simulink model "VOO _ONLY"  (R2022b)
settings: Solver=FixedStepAuto  StartTime=0.0  StopTime=10.0  FixedStep=1e-3  RelTol=1e-3  EnableMultiTasking=on
undefined symbols (not defined in the file): D10, D12, D2, D5, D9, PTA2, PTB9, PTC4, PTD0, PTD3
libraries: frdmk64flib x5
settings Model: ExtModeTrigDuration=5  Creator=aldenluscher  LastModifiedBy=aldenluscher
settings OptimizationCC: EnhancedBackFolding=on  PassReuseOutputArgsAs=Individual arguments  ZeroExternalMemoryAtStartup=off  ZeroInternalMemoryAtStartup=off  MaxStackSize=64  OptimizeBlockOrder=speed  DifferentSizesBufferReuse=on  OptimizationCustomize=off  EfficientTunableParamExpr=on
settings DebuggingCC: ParameterTunabilityLossMsg=error
settings HardwareCC: ProdBitPerPointer=32  ProdBitPerSizeT=32  ProdBitPerPtrDiffT=32  ProdLargestAtomicInteger=Long  ProdLargestAtomicFloat=Double  ProdWordSize=32  ProdHWDeviceType=ARM Compatible->ARM Cortex
settings SFSimCC: MATLABDynamicMemAlloc=off
settings RTWCC: Description=Embedded Coder  SystemTargetFile=ert.tlc  HardwareBoard=NXP FRDM-K64F  TLCOptions="-aInlineSetEventsForThisBaseRateFcn=TLC_FALSE -aSuppressMultiTaskScheduler=TLC_FALSE  -aRateBasedStepFcn=0"  TemplateMakefile=ert_default_tmf  Toolchain=GNU Tools for ARM Embedded Processors
settings CodeAppCC: ForceParamTrailComments=on  IgnoreCustomStorageClasses=off  OperatorAnnotations=on  SimulinkDataObjDesc=on  SFDataObjDesc=on  InsertBlockDesc=on
settings ERTTargetCC: ExtModeTransport=4  ExtModeMexFile=sendToCommService

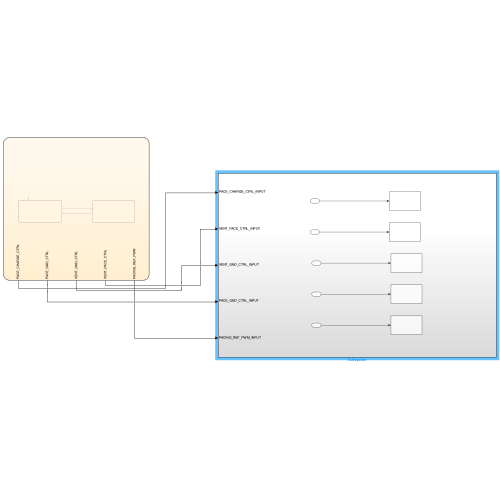
[thumbnail: Simulink's stored preview of the top-level diagram]
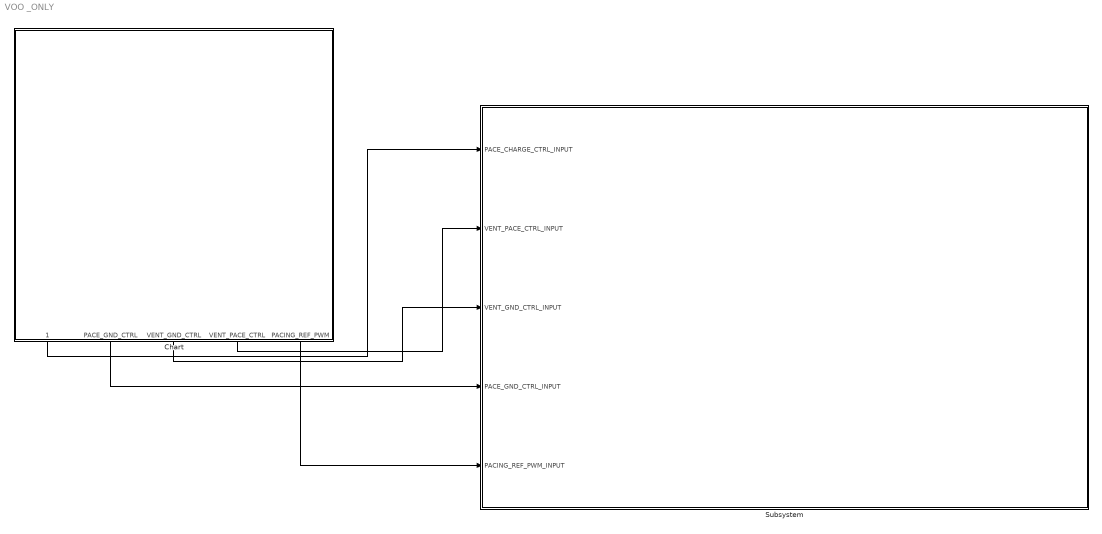
== system VOO _ONLY ==
  Chart : Stateflow chart  TreatAsAtomicUnit=on
      settings: PortSchema="{\"entries\":[{\"content\":{\"sides\":[{\"content\":{\"connectorIds\":[]},\"type\":\"ConnectorPlacement.EquallySpacedRectSide\",\"uuid\":\"ab30f6e3-f4a9-4bd5-815e-4ef92b766934\"},{\"content\":{\"connectorIds\":[],\"side\":\"RIGHT\"},\"type\":\"ConnectorPlacement.EquallySpacedRectSide\",\"uuid\":\"1d0d5e4f-590d-4361-90fd-546c5207ab80\"},{\"content\":{\"connectorIds\":[],\"side\":\"TOP\"},\"type\":\"ConnectorPlacement.EquallySpacedRectSide\",\"uuid\":\"49517801-e549-4c52-be80-c1c6727c26aa\"},{\"content\":{\"connectorIds\":[\"Out1\",\"Out2\",\"Out3\",\"Out4\",\"Out5\"],\"side\":\"BOTTOM\"},\"type\":\"ConnectorPlacement.EquallySpacedRectSide\",\"uuid\":\"3a20310d-7367-4e60-a663-7e5c4f14e519\"}]},\"type\":\"ConnectorPlacement.EquallySpacedConnector\",\"uuid\":\"1ff6ee75-2732-4076-aa82-0b614a2ae219\"}],\"packageUris\":[\"http://schema.mathworks.com/mf0/Connector/R2020b\"],\"version\":\"1.0\"}"
  Subsystem : Subsystem
  wires:
  Chart/5(PACING_REF_PWM) -> Subsystem/5(PACING_REF_PWM_INPUT)
  Chart/4(VENT_PACE_CTRL) -> Subsystem/2(VENT_PACE_CTRL_INPUT)
  Chart/3(VENT_GND_CTRL) -> Subsystem/3(VENT_GND_CTRL_INPUT)
  Chart/2(PACE_GND_CTRL) -> Subsystem/4(PACE_GND_CTRL_INPUT)
  Chart/1(PACE_CHARGE_CTRL) -> Subsystem/1(PACE_CHARGE_CTRL_INPUT)

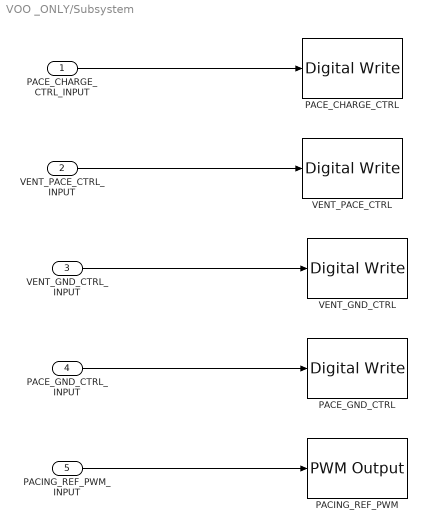
== system VOO _ONLY/Subsystem ==
  PACE_CHARGE_CTRL_INPUT : Inport
  VENT_PACE_CTRL_INPUT : Inport  Port=2
  VENT_GND_CTRL_INPUT : Inport  Port=3
  PACE_GND_CTRL_INPUT : Inport  Port=4
  PACING_REF_PWM_INPUT : Inport  Port=5
  PACE_CHARGE_CTRL : frdmk64flib/Digital Write  Whichpin=PTB9 (D2)
  PACE_GND_CTRL : frdmk64flib/Digital Write  Whichpin=PTD0 (D10)
  PACING_REF_PWM : frdmk64flib/PWM Output  Whichpin=PTA2 (D5)  InitialFrequency=2000  InitialDutyCycle=0
  VENT_GND_CTRL : frdmk64flib/Digital Write  Whichpin=PTD3 (D12)
  VENT_PACE_CTRL : frdmk64flib/Digital Write  Whichpin=PTC4 (D9)
  wires:
  VENT_PACE_CTRL_INPUT/1 -> VENT_PACE_CTRL/1
  PACE_GND_CTRL_INPUT/1 -> PACE_GND_CTRL/1
  PACE_CHARGE_CTRL_INPUT/1 -> PACE_CHARGE_CTRL/1
  PACING_REF_PWM_INPUT/1 -> PACING_REF_PWM/1
  VENT_GND_CTRL_INPUT/1 -> VENT_GND_CTRL/1

== stateflow chart VOO _ONLY/Chart ==
  state Discharging_
    PACING_REF_PWM = 60;
    PACE_CHARGE_CTRL = 1;
    PACE_GND_CTRL = 1;
    VENT_GND_CTRL = 1;
    VENT_PACE_CTRL = 0;
  state Pacing_
    PACE_CHARGE_CTRL = 0;
    PACE_GND_CTRL = 1;
    VENT_GND_CTRL = 0;
    VENT_PACE_CTRL = 1;
  (default) -> Pacing_
  Pacing_ -> Discharging_ : after(100,msec)
  Discharging_ -> Pacing_ : after(1000,msec)
  data: PACE_CHARGE_CTRL output; PACE_GND_CTRL output; VENT_GND_CTRL output; VENT_PACE_CTRL output; PACING_REF_PWM output
